simulink model "Sim4_LCL_L_comp"  (R2020b)
settings: Solver=ode1  StartTime=0.0  StopTime=3  FixedStep=Time_Step  MaxStep=1e-4  RelTol=1e-3
undefined symbols (not defined in the file): C_line, GRD00_Lg, GRD00_Rg, Theta0, Time_Step, Ug, V0, VSC01_id0
libraries: powerlib x49, Control_Lib x11, simulink x8, powerlib_meascontrol x4
(part 3 of 3)

== system Sim4_LCL_L_comp/2-Level LCL-filter/Control loops/Direct AC Voltage control/Current Limitation ==
  note: Current limitation
  Vm_dq* : Inport
  Is_dq : Inport  Port=2
  Eg_dq : Inport  Port=3
  Constant : Constant  Value=I_max_pu
  Current control : Subsystem
  Demux : Demux  Outputs=2
  Demux2 : Demux  Outputs=2
  Inverse Current control : Subsystem
  Mux : Mux  Inputs=2
  Product{,1..3} (4 alike) : Product
  Saturation Dynamic : simulink/Discontinuities/Saturation Dynamic  OutMin=[]  OutMax=[]  OutDataTypeStr=Inherit: Same as second input  OutDataType=fixdt(1, 16)  OutScaling=2^-10  DoSatur=off
  Sqrt : Sqrt  SaturateOnIntegerOverflow=on
  Sum : Sum
  Trigonometric Function : Trigonometry  Operator=atan2  NumberOfIterations=5  OutputSignalType=real
  Trigonometric Function1 : Trigonometry  Operator=cos
  Trigonometric Function2 : Trigonometry
  w_set1 : Constant
  w_set2 : Constant
  w_set3 : Constant  Value=0
  Vm_dq_sat : Outport  VectorParamsAs1DForOutWhenUnconnected=off
  wires:
  w_set3/1 -> Saturation Dynamic/3
  Constant/1 -> Saturation Dynamic/1
  Mux/1 -> Current control/1(Ig_dq0*)
  Product/1 -> Mux/1
  Demux/1 -> Product1/1, Product1/2
  Demux/2 -> Product2/1, Product2/2
  Trigonometric Function2/1 -> Product3/2
  Product2/1 -> Sum/2
  Trigonometric Function1/1 -> Product/2
  Demux2/1 -> Trigonometric Function/2
  Trigonometric Function/1 -> Trigonometric Function2/1, Trigonometric Function1/1
  Saturation Dynamic/1 -> Product/1, Product3/1
  Product1/1 -> Sum/1
  Sqrt/1 -> Saturation Dynamic/2
  Demux2/2 -> Trigonometric Function/1
  Inverse Current control/1(Is_dq*) -> Demux2/1, Demux/1
  Sum/1 -> Sqrt/1
  Product3/1 -> Mux/2
  Is_dq/1 -> Inverse Current control/2(Is_dq), Current control/2(Is_dq0)
  w_set1/1 -> Inverse Current control/4(w)
  w_set2/1 -> Current control/4(w)
  Eg_dq/1 -> Current control/3(vpcc_dq0), Inverse Current control/3(Eg_dq)
  Vm_dq*/1 -> Inverse Current control/1(Vm_dq*)
  Current control/1(vm) -> Vm_dq_sat/1

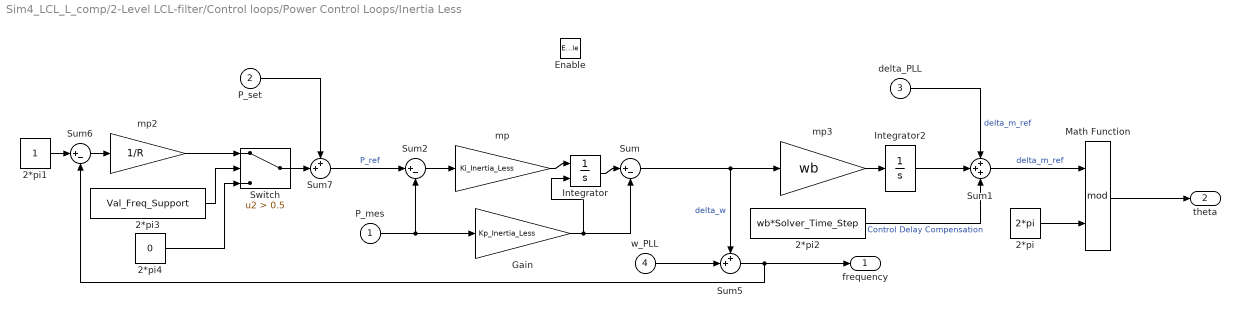
== system Sim4_LCL_L_comp/2-Level LCL-filter/Control loops/Power Control Loops/Inertia Less ==
  P_mes : Inport
  P_set : Inport  Port=2
  delta_PLL : Inport  Port=3
  w_PLL : Inport  Port=4
  Enable : EnablePort
  2*pi : Constant  Value=2*pi
  2*pi1 : Constant
  2*pi2 : Constant  Value=wb*Solver_Time_Step
  2*pi3 : Constant  Value=Val_Freq_Support
  2*pi4 : Constant  Value=0
  Gain : Gain  Gain=Kp_Inertia_Less
  Integrator : Integrator  InitialConditionSource=external
  Integrator2 : Integrator  InitialCondition=(Theta_m0)*pi/180-Theta0*pi/180
  Math Function : Math  Operator=mod  SignedPower=on  SaturateOnIntegerOverflow=on
  Sum : Sum  Inputs=|+-
  Sum1 : Sum  Inputs=+++
  Sum2 : Sum  Inputs=|+-
  Sum5 : Sum  Inputs=++|
  Sum6 : Sum  Inputs=|+-
  Sum7 : Sum  Inputs=++|
  Switch : Switch  Criteria=u2 > Threshold  Threshold=0.5
  mp : Gain  Gain=Ki_Inertia_Less
  mp2 : Gain  Gain=1/R
  mp3 : Gain  Gain=wb
  frequency : Outport  VectorParamsAs1DForOutWhenUnconnected=off
  theta : Outport  Port=2  VectorParamsAs1DForOutWhenUnconnected=off
  wires:
  Sum2/1 -> mp/1
  Sum1/1 -> Math Function/1  "delta_m_ref"
  2*pi/1 -> Math Function/2
  2*pi1/1 -> Sum6/1
  Sum6/1 -> mp2/1
  P_set/1 -> Sum7/1
  Sum7/1 -> Sum2/1  "P_ref"
  P_mes/1 -> Gain/1, Sum2/2
  Switch/1 -> Sum7/2
  Math Function/1 -> theta/1
  Sum/1 -> mp3/1, Sum5/1  "delta_w"
  mp3/1 -> Integrator2/1
  mp/1 -> Integrator/1
  delta_PLL/1 -> Sum1/1  "delta_m_ref"
  w_PLL/1 -> Sum5/2
  Sum5/1 -> frequency/1, Sum6/2
  2*pi2/1 -> Sum1/3  "Control Delay Compensation"
  Integrator2/1 -> Sum1/2
  mp2/1 -> Switch/1
  2*pi3/1 -> Switch/2
  2*pi4/1 -> Switch/3
  Integrator/1 -> Sum/1
  Gain/1 -> Integrator/2, Sum/2

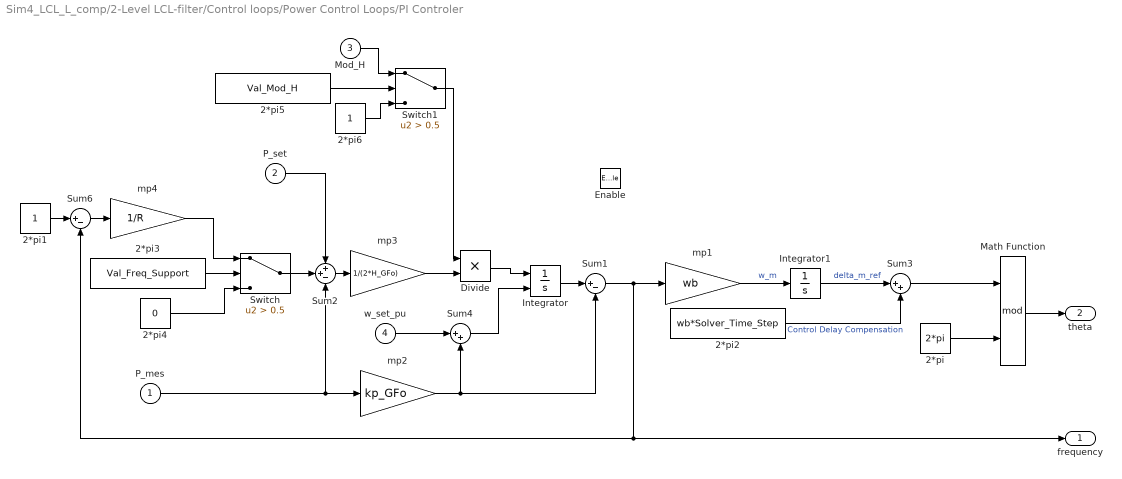
== system Sim4_LCL_L_comp/2-Level LCL-filter/Control loops/Power Control Loops/PI Controler ==
  P_mes : Inport
  P_set : Inport  Port=2
  Mod_H : Inport  Port=3
  w_set_pu : Inport  Port=4
  Enable : EnablePort
  2*pi : Constant  Value=2*pi
  2*pi1 : Constant
  2*pi2 : Constant  Value=wb*Solver_Time_Step
  2*pi3 : Constant  Value=Val_Freq_Support
  2*pi4 : Constant  Value=0
  2*pi5 : Constant  Value=Val_Mod_H
  2*pi6 : Constant
  Divide : Product  Inputs=**
  Integrator : Integrator  InitialConditionSource=external
  Integrator1 : Integrator  InitialCondition=(Theta_m0)*pi/180
  Math Function : Math  Operator=mod  SignedPower=on  SaturateOnIntegerOverflow=on
  Sum1 : Sum  Inputs=|+-
  Sum2 : Sum  Inputs=++-
  Sum3 : Sum  Inputs=|++
  Sum4 : Sum  Inputs=|++
  Sum6 : Sum  Inputs=|+-
  Switch : Switch  Criteria=u2 > Threshold  Threshold=0.5
  Switch1 : Switch  Criteria=u2 > Threshold  Threshold=0.5
  mp1 : Gain  Gain=wb
  mp2 : Gain  Gain=kp_GFo
  mp3 : Gain  Gain=1/(2*H_GFo)
  mp4 : Gain  Gain=1/R
  frequency : Outport  VectorParamsAs1DForOutWhenUnconnected=off
  theta : Outport  Port=2  VectorParamsAs1DForOutWhenUnconnected=off
  wires:
  Sum2/1 -> mp3/1
  Integrator1/1 -> Sum3/1  "delta_m_ref"
  Math Function/1 -> theta/1
  2*pi/1 -> Math Function/2
  w_set_pu/1 -> Sum4/1
  P_set/1 -> Sum2/1
  Integrator/1 -> Sum1/1
  Sum1/1 -> mp1/1, frequency/1, Sum6/2
  mp1/1 -> Integrator1/1  "w_m"
  Sum3/1 -> Math Function/1
  2*pi2/1 -> Sum3/2  "Control Delay Compensation"
  P_mes/1 -> Sum2/3, mp2/1
  mp2/1 -> Sum1/2, Sum4/2
  mp3/1 -> Divide/2
  Sum4/1 -> Integrator/2
  mp4/1 -> Switch/1
  2*pi1/1 -> Sum6/1
  2*pi3/1 -> Switch/2
  Sum6/1 -> mp4/1
  2*pi4/1 -> Switch/3
  Switch/1 -> Sum2/2
  2*pi5/1 -> Switch1/2
  2*pi6/1 -> Switch1/3
  Mod_H/1 -> Switch1/1
  Divide/1 -> Integrator/1
  Switch1/1 -> Divide/1

== system Sim4_LCL_L_comp/2-Level LCL-filter/Control loops/Power Control Loops/Subsystem ==
  Delta_E_dq : Inport
  Constant : Constant
  Constant1 : Constant  Value=2
  Delay : Delay  DelayLength=1  InitialCondition=1
  Demux : Demux  Outputs=2
  Pow : Math  Operator=pow  SignedPower=on  RndMeth=Zero  SaturateOnIntegerOverflow=on
  Square : Math  Operator=square  SignedPower=on  RndMeth=Zero  SaturateOnIntegerOverflow=on
  Square1 : Math  Operator=square  SignedPower=on  RndMeth=Zero  SaturateOnIntegerOverflow=on
  Sum : Sum  Inputs=|+-
  Sum5 : Sum
  Mod_h : Outport  VectorParamsAs1DForOutWhenUnconnected=off
  wires:
  Delta_E_dq/1 -> Delay/1
  Square/1 -> Sum5/1
  Pow/1 -> Mod_h/1
  Constant1/1 -> Pow/2
  Demux/2 -> Square1/1
  Constant/1 -> Sum/1
  Sum5/1 -> Pow/1
  Square1/1 -> Sum5/2
  Demux/1 -> Sum/2
  Sum/1 -> Square/1
  Delay/1 -> Demux/1

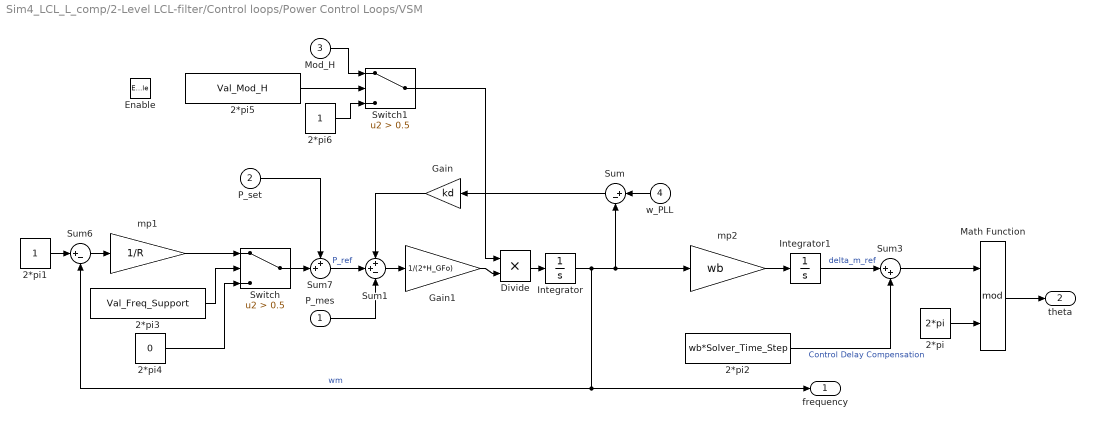
== system Sim4_LCL_L_comp/2-Level LCL-filter/Control loops/Power Control Loops/VSM ==
  P_mes : Inport
  P_set : Inport  Port=2
  Mod_H : Inport  Port=3
  w_PLL : Inport  Port=4
  Enable : EnablePort
  2*pi : Constant  Value=2*pi
  2*pi1 : Constant
  2*pi2 : Constant  Value=wb*Solver_Time_Step
  2*pi3 : Constant  Value=Val_Freq_Support
  2*pi4 : Constant  Value=0
  2*pi5 : Constant  Value=Val_Mod_H
  2*pi6 : Constant
  Divide : Product  Inputs=**
  Gain : Gain  Gain=kd
  Gain1 : Gain  Gain=1/(2*H_GFo)
  Integrator : Integrator  InitialCondition=1
  Integrator1 : Integrator  InitialCondition=Theta_m0*pi/180
  Math Function : Math  Operator=mod  SignedPower=on  SaturateOnIntegerOverflow=on
  Sum : Sum  Inputs=|+-
  Sum1 : Sum  Inputs=++-
  Sum3 : Sum  Inputs=|++
  Sum6 : Sum  Inputs=|+-
  Sum7 : Sum  Inputs=++|
  Switch : Switch  Criteria=u2 > Threshold  Threshold=0.5
  Switch1 : Switch  Criteria=u2 > Threshold  Threshold=0.5
  mp1 : Gain  Gain=1/R
  mp2 : Gain  Gain=wb
  frequency : Outport  VectorParamsAs1DForOutWhenUnconnected=off
  theta : Outport  Port=2  VectorParamsAs1DForOutWhenUnconnected=off
  wires:
  2*pi/1 -> Math Function/2
  Math Function/1 -> theta/1
  Integrator1/1 -> Sum3/1  "delta_m_ref"
  Integrator/1 -> Sum/2, mp2/1, frequency/1, Sum6/2  "wm"
  P_mes/1 -> Sum1/3
  mp2/1 -> Integrator1/1
  2*pi2/1 -> Sum3/2  "Control Delay Compensation"
  Sum3/1 -> Math Function/1
  Switch/1 -> Sum7/2
  P_set/1 -> Sum7/1
  Sum6/1 -> mp1/1
  2*pi1/1 -> Sum6/1
  mp1/1 -> Switch/1
  2*pi3/1 -> Switch/2
  2*pi4/1 -> Switch/3
  w_PLL/1 -> Sum/1
  Sum/1 -> Gain/1
  Gain/1 -> Sum1/1
  Sum1/1 -> Gain1/1
  Sum7/1 -> Sum1/2  "P_ref"
  2*pi5/1 -> Switch1/2
  2*pi6/1 -> Switch1/3
  Mod_H/1 -> Switch1/1
  Divide/1 -> Integrator/1
  Gain1/1 -> Divide/2
  Switch1/1 -> Divide/1

== system Sim4_LCL_L_comp/2-Level LCL-filter/Control loops/Transient Damping Resistance/Filter w_LF ==
  e : Inport
  1/T_LP : Gain  Gain=W_TVR  SaturateOnIntegerOverflow=on  OutDataTypeStr=Inherit: Same as input  ParamDataTypeStr=Inherit: Same as input
  Integrator : Integrator  InitialConditionSource=external  InitialCondition=[VSC01_id0*0.04]
  Sum1 : Sum  Inputs=|+-  InputSameDT=on  SaturateOnIntegerOverflow=on  OutDataTypeStr=Inherit: Same as first input
  s : Outport  VectorParamsAs1DForOutWhenUnconnected=off
  wires:
  e/1 -> Sum1/1, Integrator/2
  Integrator/1 -> s/1, Sum1/2
  1/T_LP/1 -> Integrator/1
  Sum1/1 -> 1/T_LP/1

== system Sim4_LCL_L_comp/2-Level LCL-filter/Control loops/VI/dq to phasor ==
  dq_mes : Inport
  Demux : Demux  Outputs=2
      settings: DisplayOption=none
  Sqrt : Sqrt  SaturateOnIntegerOverflow=on
  Sum4 : Sum  Inputs=|++  InputSameDT=on  SaturateOnIntegerOverflow=on  OutDataTypeStr=Inherit: Same as first input
  Vrdird : Product  InputSameDT=on  RndMeth=Zero  SaturateOnIntegerOverflow=on  OutDataTypeStr=Inherit: Same as first input
  Vrqirq : Product  InputSameDT=on  RndMeth=Zero  SaturateOnIntegerOverflow=on  OutDataTypeStr=Inherit: Same as first input
  rms : Outport  VectorParamsAs1DForOutWhenUnconnected=off
  wires:
  Sum4/1 -> Sqrt/1
  Vrqirq/1 -> Sum4/2
  Vrdird/1 -> Sum4/1
  Demux/2 -> Vrqirq/2, Vrqirq/1
  Demux/1 -> Vrdird/2, Vrdird/1
  dq_mes/1 -> Demux/1
  Sqrt/1 -> rms/1

== system Sim4_LCL_L_comp/VSC_average/Control loops/Current Limitation/Current control ==
  Ig_dq0* : Inport
  Ig_dq0 : Inport  Port=2
  vg_dq0 : Inport  Port=3
  w : Inport  Port=4
  Demux : Demux  Outputs=2
  Demux1 : Demux  Outputs=2
  Demux2 : Demux  Outputs=2
  Gain Corrector : Gain  Gain=3/(Tr_I_max/1000)*Lt_pu
  Gain Corrector1 : Gain  Gain=3/(Tr_I_max/1000)*Lt_pu
  Mux : Mux  Inputs=2
  Product : Product  RndMeth=Zero
  Product1 : Product  RndMeth=Zero
  Sum : Sum  Inputs=|+-
  Sum2 : Sum  Inputs=|+-
  Sum3 : Sum  Inputs=|++
  Sum5 : Sum  Inputs=++|
  Sum6 : Sum  Inputs=-+|
  Sum7 : Sum  Inputs=++|
  vpcc_abc{1,3..6} (5 alike) : Scope
  w*Lf_pu : Gain  Gain=Lt_pu
  vm : Outport  InitialOutput=0  VectorParamsAs1DForOutWhenUnconnected=off
  wires:
  Demux2/2 -> Sum7/1
  Demux2/1 -> Sum3/2
  w/1 -> vpcc_abc5/1, w*Lf_pu/1
  Sum/1 -> vpcc_abc1/1, Gain Corrector/1
  Sum7/1 -> Mux/2  "Vm_q*"
  Sum3/1 -> Mux/1, vpcc_abc3/1  "Vm_d*"
  Sum5/1 -> Sum7/2
  Product1/1 -> Sum5/1
  Gain Corrector1/1 -> Sum5/2
  Demux/2 -> Sum6/2
  Sum2/1 -> Sum3/1
  Product/1 -> Sum2/2
  Demux1/2 -> Sum6/1, Product/1
  w*Lf_pu/1 -> Product/2, Product1/1
  Gain Corrector/1 -> Sum2/1
  Demux1/1 -> Sum/2, Product1/2
  Demux/1 -> Sum/1
  Ig_dq0/1 -> Demux1/1
  vg_dq0/1 -> Demux2/1, vpcc_abc6/1
  Sum6/1 -> Gain Corrector1/1
  Ig_dq0*/1 -> vpcc_abc4/1, Demux/1
  Mux/1 -> vm/1

== system Sim4_LCL_L_comp/VSC_average/Control loops/Current Limitation/Inverse Current control ==
  Vm_dq* : Inport
  Ig_dq : Inport  Port=2
  vg_dq : Inport  Port=3
  w : Inport  Port=4
  Demux : Demux  Outputs=2
  Demux1 : Demux  Outputs=2
  Demux2 : Demux  Outputs=2
  Gain Corrector2 : Gain  Gain=1/(3/(Tr_I_max/1000)*Lt_pu)
  Gain Corrector3 : Gain  Gain=1/(3/(Tr_I_max/1000)*Lt_pu)
  Mux : Mux  Inputs=2
  Product : Product  RndMeth=Zero
  Product1 : Product  RndMeth=Zero
  Sum : Sum  Inputs=|+-
  Sum2 : Sum  Inputs=|++
  Sum3 : Sum  Inputs=|++
  Sum5 : Sum  Inputs=-+|
  Sum6 : Sum  Inputs=-+|
  Sum7 : Sum  Inputs=++|
  w*Lf_pu : Gain  Gain=Lt_pu
  Is_dq* : Outport  InitialOutput=0  VectorParamsAs1DForOutWhenUnconnected=off
  wires:
  vg_dq/1 -> Demux2/1
  Ig_dq/1 -> Demux1/1
  Vm_dq*/1 -> Demux/1
  Demux/1 -> Sum/1
  Demux1/1 -> Sum3/2, Product1/2
  Sum/1 -> Sum2/1
  w*Lf_pu/1 -> Product1/1, Product/2
  Product/1 -> Sum2/2
  Sum2/1 -> Gain Corrector3/1
  Mux/1 -> Is_dq*/1
  Demux/2 -> Sum6/2
  Sum6/1 -> Sum5/2
  Sum5/1 -> Gain Corrector2/1
  Sum3/1 -> Mux/1  "is_d*"
  Sum7/1 -> Mux/2  "is_q*"
  w/1 -> w*Lf_pu/1
  Demux1/2 -> Sum7/1, Product/1
  Gain Corrector3/1 -> Sum3/1
  Demux2/1 -> Sum/2
  Demux2/2 -> Sum6/1
  Product1/1 -> Sum5/1
  Gain Corrector2/1 -> Sum7/2

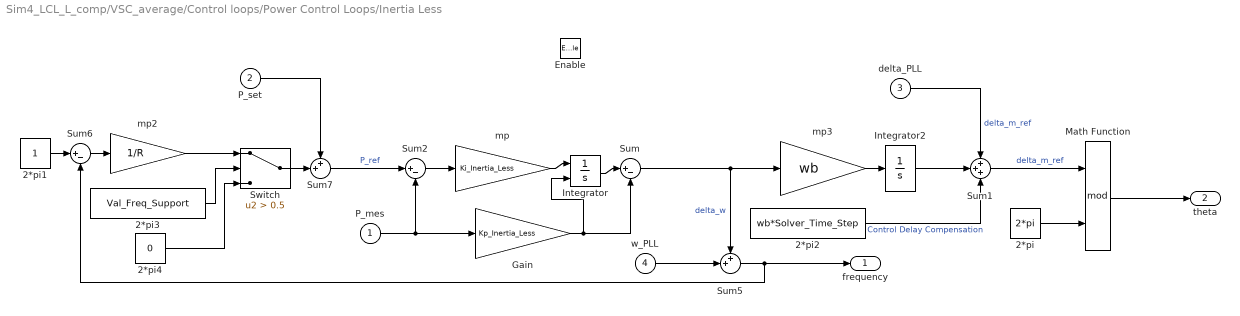
== system Sim4_LCL_L_comp/VSC_average/Control loops/Power Control Loops/Inertia Less ==
  P_mes : Inport
  P_set : Inport  Port=2
  delta_PLL : Inport  Port=3
  w_PLL : Inport  Port=4
  Enable : EnablePort
  2*pi : Constant  Value=2*pi
  2*pi1 : Constant
  2*pi2 : Constant  Value=wb*Solver_Time_Step
  2*pi3 : Constant  Value=Val_Freq_Support
  2*pi4 : Constant  Value=0
  Gain : Gain  Gain=Kp_Inertia_Less
  Integrator : Integrator  InitialConditionSource=external
  Integrator2 : Integrator  InitialCondition=(Theta_vsc0)*pi/180-Theta0*pi/180
  Math Function : Math  Operator=mod  SignedPower=on  SaturateOnIntegerOverflow=on
  Sum : Sum  Inputs=|+-
  Sum1 : Sum  Inputs=+++
  Sum2 : Sum  Inputs=|+-
  Sum5 : Sum  Inputs=++|
  Sum6 : Sum  Inputs=|+-
  Sum7 : Sum  Inputs=++|
  Switch : Switch  Criteria=u2 > Threshold  Threshold=0.5
  mp : Gain  Gain=Ki_Inertia_Less
  mp2 : Gain  Gain=1/R
  mp3 : Gain  Gain=wb
  frequency : Outport  VectorParamsAs1DForOutWhenUnconnected=off
  theta : Outport  Port=2  VectorParamsAs1DForOutWhenUnconnected=off
  wires:
  Gain/1 -> Sum/2, Integrator/2
  Integrator/1 -> Sum/1
  2*pi4/1 -> Switch/3
  2*pi3/1 -> Switch/2
  mp2/1 -> Switch/1
  Integrator2/1 -> Sum1/2
  2*pi2/1 -> Sum1/3  "Control Delay Compensation"
  Sum5/1 -> Sum6/2, frequency/1
  w_PLL/1 -> Sum5/2
  delta_PLL/1 -> Sum1/1  "delta_m_ref"
  mp/1 -> Integrator/1
  mp3/1 -> Integrator2/1
  Sum/1 -> Sum5/1, mp3/1  "delta_w"
  Math Function/1 -> theta/1
  Switch/1 -> Sum7/2
  P_mes/1 -> Sum2/2, Gain/1
  Sum7/1 -> Sum2/1  "P_ref"
  P_set/1 -> Sum7/1
  Sum6/1 -> mp2/1
  2*pi1/1 -> Sum6/1
  2*pi/1 -> Math Function/2
  Sum1/1 -> Math Function/1  "delta_m_ref"
  Sum2/1 -> mp/1

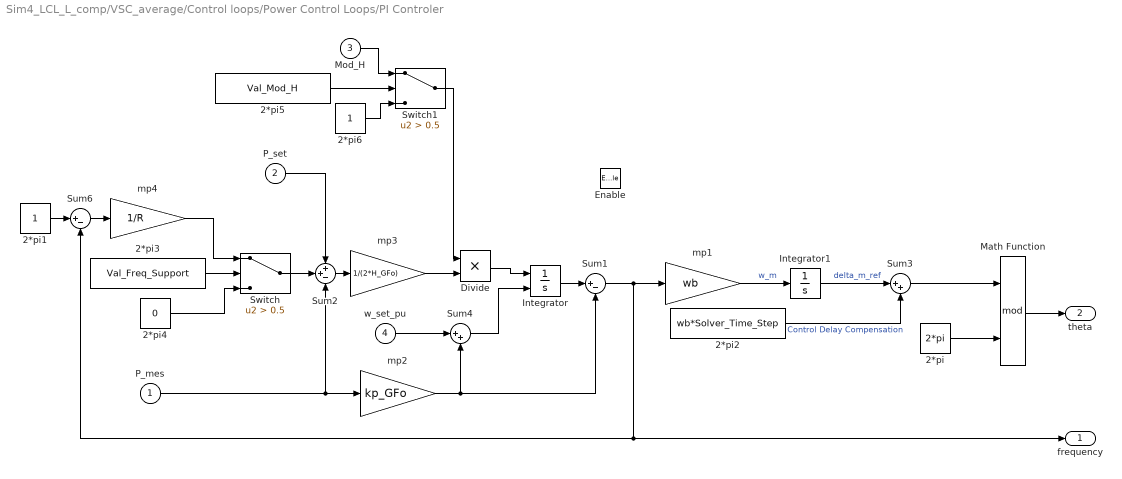
== system Sim4_LCL_L_comp/VSC_average/Control loops/Power Control Loops/PI Controler ==
  P_mes : Inport
  P_set : Inport  Port=2
  Mod_H : Inport  Port=3
  w_set_pu : Inport  Port=4
  Enable : EnablePort
  2*pi : Constant  Value=2*pi
  2*pi1 : Constant
  2*pi2 : Constant  Value=wb*Solver_Time_Step
  2*pi3 : Constant  Value=Val_Freq_Support
  2*pi4 : Constant  Value=0
  2*pi5 : Constant  Value=Val_Mod_H
  2*pi6 : Constant
  Divide : Product  Inputs=**
  Integrator : Integrator  InitialConditionSource=external
  Integrator1 : Integrator  InitialCondition=(Theta_vsc0)*pi/180
  Math Function : Math  Operator=mod  SignedPower=on  SaturateOnIntegerOverflow=on
  Sum1 : Sum  Inputs=|+-
  Sum2 : Sum  Inputs=++-
  Sum3 : Sum  Inputs=|++
  Sum4 : Sum  Inputs=|++
  Sum6 : Sum  Inputs=|+-
  Switch : Switch  Criteria=u2 > Threshold  Threshold=0.5
  Switch1 : Switch  Criteria=u2 > Threshold  Threshold=0.5
  mp1 : Gain  Gain=wb
  mp2 : Gain  Gain=kp_GFo
  mp3 : Gain  Gain=1/(2*H_GFo)
  mp4 : Gain  Gain=1/R
  frequency : Outport  VectorParamsAs1DForOutWhenUnconnected=off
  theta : Outport  Port=2  VectorParamsAs1DForOutWhenUnconnected=off
  wires:
  Switch1/1 -> Divide/1
  Divide/1 -> Integrator/1
  Mod_H/1 -> Switch1/1
  2*pi6/1 -> Switch1/3
  2*pi5/1 -> Switch1/2
  Switch/1 -> Sum2/2
  2*pi4/1 -> Switch/3
  Sum6/1 -> mp4/1
  2*pi3/1 -> Switch/2
  2*pi1/1 -> Sum6/1
  mp4/1 -> Switch/1
  Sum4/1 -> Integrator/2
  mp3/1 -> Divide/2
  mp2/1 -> Sum4/2, Sum1/2
  P_mes/1 -> mp2/1, Sum2/3
  2*pi2/1 -> Sum3/2  "Control Delay Compensation"
  Sum3/1 -> Math Function/1
  mp1/1 -> Integrator1/1  "w_m"
  Sum1/1 -> Sum6/2, frequency/1, mp1/1
  Integrator/1 -> Sum1/1
  P_set/1 -> Sum2/1
  w_set_pu/1 -> Sum4/1
  2*pi/1 -> Math Function/2
  Math Function/1 -> theta/1
  Integrator1/1 -> Sum3/1  "delta_m_ref"
  Sum2/1 -> mp3/1

== system Sim4_LCL_L_comp/VSC_average/Control loops/Power Control Loops/Subsystem ==
  Delta_E_dq : Inport
  Constant : Constant
  Constant1 : Constant  Value=2
  Delay : Delay  DelayLength=1  InitialCondition=1
  Demux : Demux  Outputs=2
  Pow : Math  Operator=pow  SignedPower=on  RndMeth=Zero  SaturateOnIntegerOverflow=on
  Square : Math  Operator=square  SignedPower=on  RndMeth=Zero  SaturateOnIntegerOverflow=on
  Square1 : Math  Operator=square  SignedPower=on  RndMeth=Zero  SaturateOnIntegerOverflow=on
  Sum : Sum  Inputs=|+-
  Sum5 : Sum
  Mod_h : Outport  VectorParamsAs1DForOutWhenUnconnected=off
  wires:
  Delay/1 -> Demux/1
  Sum/1 -> Square/1
  Demux/1 -> Sum/2
  Square1/1 -> Sum5/2
  Sum5/1 -> Pow/1
  Constant/1 -> Sum/1
  Demux/2 -> Square1/1
  Constant1/1 -> Pow/2
  Pow/1 -> Mod_h/1
  Square/1 -> Sum5/1
  Delta_E_dq/1 -> Delay/1

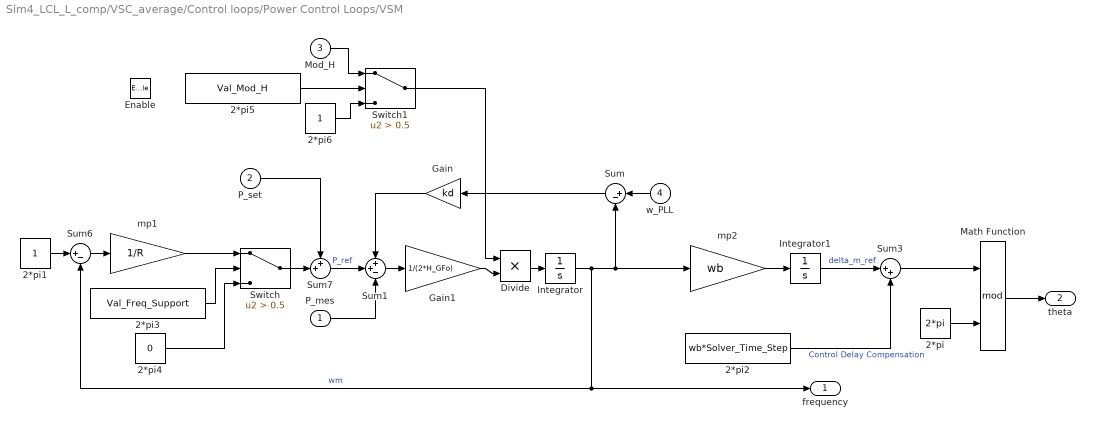
== system Sim4_LCL_L_comp/VSC_average/Control loops/Power Control Loops/VSM ==
  P_mes : Inport
  P_set : Inport  Port=2
  Mod_H : Inport  Port=3
  w_PLL : Inport  Port=4
  Enable : EnablePort
  2*pi : Constant  Value=2*pi
  2*pi1 : Constant
  2*pi2 : Constant  Value=wb*Solver_Time_Step
  2*pi3 : Constant  Value=Val_Freq_Support
  2*pi4 : Constant  Value=0
  2*pi5 : Constant  Value=Val_Mod_H
  2*pi6 : Constant
  Divide : Product  Inputs=**
  Gain : Gain  Gain=kd
  Gain1 : Gain  Gain=1/(2*H_GFo)
  Integrator : Integrator  InitialCondition=1
  Integrator1 : Integrator  InitialCondition=Theta_vsc0*pi/180
  Math Function : Math  Operator=mod  SignedPower=on  SaturateOnIntegerOverflow=on
  Sum : Sum  Inputs=|+-
  Sum1 : Sum  Inputs=++-
  Sum3 : Sum  Inputs=|++
  Sum6 : Sum  Inputs=|+-
  Sum7 : Sum  Inputs=++|
  Switch : Switch  Criteria=u2 > Threshold  Threshold=0.5
  Switch1 : Switch  Criteria=u2 > Threshold  Threshold=0.5
  mp1 : Gain  Gain=1/R
  mp2 : Gain  Gain=wb
  frequency : Outport  VectorParamsAs1DForOutWhenUnconnected=off
  theta : Outport  Port=2  VectorParamsAs1DForOutWhenUnconnected=off
  wires:
  Switch1/1 -> Divide/1
  Gain1/1 -> Divide/2
  Divide/1 -> Integrator/1
  Mod_H/1 -> Switch1/1
  2*pi6/1 -> Switch1/3
  2*pi5/1 -> Switch1/2
  Sum7/1 -> Sum1/2  "P_ref"
  Sum1/1 -> Gain1/1
  Gain/1 -> Sum1/1
  Sum/1 -> Gain/1
  w_PLL/1 -> Sum/1
  2*pi4/1 -> Switch/3
  2*pi3/1 -> Switch/2
  mp1/1 -> Switch/1
  2*pi1/1 -> Sum6/1
  Sum6/1 -> mp1/1
  P_set/1 -> Sum7/1
  Switch/1 -> Sum7/2
  Sum3/1 -> Math Function/1
  2*pi2/1 -> Sum3/2  "Control Delay Compensation"
  mp2/1 -> Integrator1/1
  P_mes/1 -> Sum1/3
  Integrator/1 -> Sum6/2, frequency/1, mp2/1, Sum/2  "wm"
  Integrator1/1 -> Sum3/1  "delta_m_ref"
  Math Function/1 -> theta/1
  2*pi/1 -> Math Function/2

== system Sim4_LCL_L_comp/VSC_average/Control loops/Transient Damping Resistance/Filter w_LF ==
  e : Inport
  1/T_LP : Gain  Gain=W_TVR  SaturateOnIntegerOverflow=on  OutDataTypeStr=Inherit: Same as input  ParamDataTypeStr=Inherit: Same as input
  Integrator : Integrator  InitialConditionSource=external  InitialCondition=[VSC01_id0*0.04]
  Sum1 : Sum  Inputs=|+-  InputSameDT=on  SaturateOnIntegerOverflow=on  OutDataTypeStr=Inherit: Same as first input
  s : Outport  VectorParamsAs1DForOutWhenUnconnected=off
  wires:
  e/1 -> Sum1/1, Integrator/2
  Integrator/1 -> s/1, Sum1/2
  1/T_LP/1 -> Integrator/1
  Sum1/1 -> 1/T_LP/1

== system Sim4_LCL_L_comp/VSC_average/Control loops/VI/dq to phasor ==
  dq_mes : Inport
  Demux : Demux  Outputs=2
      settings: DisplayOption=none
  Sqrt : Sqrt  SaturateOnIntegerOverflow=on
  Sum4 : Sum  Inputs=|++  InputSameDT=on  SaturateOnIntegerOverflow=on  OutDataTypeStr=Inherit: Same as first input
  Vrdird : Product  InputSameDT=on  RndMeth=Zero  SaturateOnIntegerOverflow=on  OutDataTypeStr=Inherit: Same as first input
  Vrqirq : Product  InputSameDT=on  RndMeth=Zero  SaturateOnIntegerOverflow=on  OutDataTypeStr=Inherit: Same as first input
  rms : Outport  VectorParamsAs1DForOutWhenUnconnected=off
  wires:
  Sum4/1 -> Sqrt/1
  Vrqirq/1 -> Sum4/2
  Vrdird/1 -> Sum4/1
  Demux/2 -> Vrqirq/2, Vrqirq/1
  Demux/1 -> Vrdird/2, Vrdird/1
  dq_mes/1 -> Demux/1
  Sqrt/1 -> rms/1

== system Sim4_LCL_L_comp/2-Level LCL-filter/Control loops/Direct AC Voltage control/Current Limitation/Current control ==
  Ig_dq0* : Inport
  Is_dq0 : Inport  Port=2
  vpcc_dq0 : Inport  Port=3
  w : Inport  Port=4
  Demux : Demux  Outputs=2
  Demux1 : Demux  Outputs=2
  Demux2 : Demux  Outputs=2
  Gain Corrector : Gain  Gain=3/(Tr_I_max/1000)*Lf_pu
  Gain Corrector1 : Gain  Gain=3/(Tr_I_max/1000)*Lf_pu
  Mux : Mux  Inputs=2
  Product : Product  RndMeth=Zero
  Product1 : Product  RndMeth=Zero
  Sum : Sum  Inputs=|+-
  Sum2 : Sum  Inputs=|+-
  Sum3 : Sum  Inputs=|++
  Sum5 : Sum  Inputs=++|
  Sum6 : Sum  Inputs=-+|
  Sum7 : Sum  Inputs=++|
  vpcc_abc{1,3..6} (5 alike) : Scope
  w*Lf_pu : Gain  Gain=Lf_pu
  vm : Outport  InitialOutput=0  VectorParamsAs1DForOutWhenUnconnected=off
  wires:
  Demux2/2 -> Sum7/1
  Demux2/1 -> Sum3/2
  w/1 -> vpcc_abc5/1, w*Lf_pu/1
  Sum/1 -> vpcc_abc1/1, Gain Corrector/1
  Sum7/1 -> Mux/2  "Vm_q*"
  Sum3/1 -> Mux/1, vpcc_abc3/1  "Vm_d*"
  Sum5/1 -> Sum7/2
  Product1/1 -> Sum5/1
  Gain Corrector1/1 -> Sum5/2
  Demux/2 -> Sum6/2
  Sum2/1 -> Sum3/1
  Product/1 -> Sum2/2
  Demux1/2 -> Sum6/1, Product/1
  w*Lf_pu/1 -> Product/2, Product1/1
  Gain Corrector/1 -> Sum2/1
  Demux1/1 -> Sum/2, Product1/2
  Demux/1 -> Sum/1
  Is_dq0/1 -> Demux1/1
  vpcc_dq0/1 -> Demux2/1, vpcc_abc6/1
  Sum6/1 -> Gain Corrector1/1
  Ig_dq0*/1 -> vpcc_abc4/1, Demux/1
  Mux/1 -> vm/1

== system Sim4_LCL_L_comp/2-Level LCL-filter/Control loops/Direct AC Voltage control/Current Limitation/Inverse Current control ==
  Vm_dq* : Inport
  Is_dq : Inport  Port=2
  Eg_dq : Inport  Port=3
  w : Inport  Port=4
  Demux : Demux  Outputs=2
  Demux1 : Demux  Outputs=2
  Demux2 : Demux  Outputs=2
  Gain Corrector2 : Gain  Gain=1/(3/(Tr_I_max/1000)*Lf_pu)
  Gain Corrector3 : Gain  Gain=1/(3/(Tr_I_max/1000)*Lf_pu)
  Mux : Mux  Inputs=2
  Product : Product  RndMeth=Zero
  Product1 : Product  RndMeth=Zero
  Sum : Sum  Inputs=|+-
  Sum2 : Sum  Inputs=|++
  Sum3 : Sum  Inputs=|++
  Sum5 : Sum  Inputs=-+|
  Sum6 : Sum  Inputs=-+|
  Sum7 : Sum  Inputs=++|
  w*Lf_pu : Gain  Gain=Lf_pu
  Is_dq* : Outport  InitialOutput=0  VectorParamsAs1DForOutWhenUnconnected=off
  wires:
  Eg_dq/1 -> Demux2/1
  Is_dq/1 -> Demux1/1
  Vm_dq*/1 -> Demux/1
  Demux/1 -> Sum/1
  Demux1/1 -> Sum3/2, Product1/2
  Sum/1 -> Sum2/1
  w*Lf_pu/1 -> Product1/1, Product/2
  Product/1 -> Sum2/2
  Sum2/1 -> Gain Corrector3/1
  Mux/1 -> Is_dq*/1
  Demux/2 -> Sum6/2
  Sum6/1 -> Sum5/2
  Sum5/1 -> Gain Corrector2/1
  Sum3/1 -> Mux/1  "is_d*"
  Sum7/1 -> Mux/2  "is_q*"
  w/1 -> w*Lf_pu/1
  Demux1/2 -> Sum7/1, Product/1
  Gain Corrector3/1 -> Sum3/1
  Demux2/1 -> Sum/2
  Demux2/2 -> Sum6/1
  Product1/1 -> Sum5/1
  Gain Corrector2/1 -> Sum7/2
